simulink model "attack_and_release_filter"  (R2020b)
settings: Solver=FixedStepDiscrete  StartTime=0.0  StopTime=stopTime  FixedStep=2.0833333333333333e-05  RelTol=1e-3
InitFcn:
  | initCallback
StopFcn:
  | stopCallback
undefined symbols (not defined in the file or in its folder): buf_r
libraries: simulink x1
settings Model: Creator=Ross  LastModifiedBy=conno
settings DataIOCC: SaveOutput=off  SaveTime=off  ReturnWorkspaceOutputs=off
settings OptimizationCC: BlockReduction=off  ConditionallyExecuteInputs=off  DefaultParameterBehavior=Inlined
settings DebuggingCC: ReadBeforeWriteMsg=DisableAll  WriteAfterWriteMsg=DisableAll  WriteAfterReadMsg=DisableAll  AlgebraicLoopMsg=error  MultiTaskDSMMsg=none  SingleTaskRateTransMsg=error  PregeneratedLibrarySubsystemCodeDiagnostic=none  ArithmeticOperatorsInVariantConditions=warning
settings HardwareCC: ProdBitPerPointer=32  ProdBitPerSizeT=32  ProdBitPerPtrDiffT=32  ProdLargestAtomicFloat=None  ProdIntDivRoundTo=Undefined  ProdEndianess=Unspecified  ProdWordSize=32  ProdHWDeviceType=ASIC/FPGA->ASIC/FPGA  TargetBitPerPointer=64  TargetBitPerSizeT=64  TargetBitPerPtrDiffT=64  TargetLongLongMode=on  TargetIntDivRoundTo=Zero  TargetEndianess=LittleEndian  TargetWordSize=64  TargetHWDeviceType=Custom Processor->MATLAB Host Computer  ProdEqTarget=off
settings ModelReferenceCC: UpdateModelReferenceTargets=IfOutOfDate
settings SFSimCC: SFSimEcho=off  SimUseLocalCustomCode=off  CustomCodeUndefinedFunction=UseInterfaceOnly
settings RTWCC: RTWUseLocalCustomCode=off

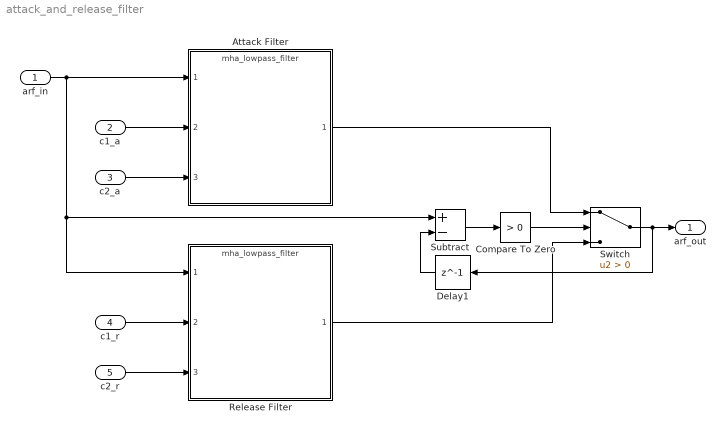
== system attack_and_release_filter ==
  arf_in : Inport  OutDataTypeStr=single  PortDimensions=1  SampleTime=[2.0833333333333333e-05,0]
  c1_a : Inport  Port=2  OutDataTypeStr=single  PortDimensions=1
  c2_a : Inport  Port=3  OutDataTypeStr=single  PortDimensions=1
  c1_r : Inport  Port=4  OutDataTypeStr=single  PortDimensions=1
  c2_r : Inport  Port=5  OutDataTypeStr=single  PortDimensions=1
  Attack Filter : ModelReference  ModelNameDialog=mha_lowpass_filter.slx  SimulationMode=Normal  ModelReferenceVersion=1.119
  Compare To Zero : simulink/Logic and Bit Operations/Compare To Zero  relop=>  OutDataTypeStr=boolean
  Delay1 : Delay  DelayLength=1  InitialCondition=0
  Release Filter : ModelReference  ModelNameDialog=mha_lowpass_filter.slx  SimulationMode=Normal  ModelReferenceVersion=1.119
  Subtract : Sum  Inputs=+-  OutDataTypeStr=Inherit: Keep MSB
  Switch : Switch  Criteria=u2 > Threshold
  arf_out : Outport  OutDataTypeStr=single  PortDimensions=1  SampleTime=[2.0833333333333333e-05,0]  InitialOutput=[buf_r(1,1)]  VectorParamsAs1DForOutWhenUnconnected=off
  wires:
  c1_a/1 -> Attack Filter/2
  arf_in/1 -> Attack Filter/1, Subtract/1, Release Filter/1
  c2_a/1 -> Attack Filter/3
  c2_r/1 -> Release Filter/3
  c1_r/1 -> Release Filter/2
  Switch/1 -> arf_out/1, Delay1/1
  Attack Filter/1 -> Switch/1
  Release Filter/1 -> Switch/3
  Subtract/1 -> Compare To Zero/1
  Compare To Zero/1 -> Switch/2
  Delay1/1 -> Subtract/2
